simulink model "Receiver"  (R2021b)
settings: Solver=FixedStepDiscrete  StartTime=0.0  StopTime=inf  RelTol=1e-3
undefined symbols (not defined in the file): D4
libraries: androiduilib x4, androidcommunicationlib x1
settings Model: Creator=Nishikant Parmar  LastModifiedBy=Nishikant Parmar
settings OptimizationCC: EnhancedBackFolding=on  PassReuseOutputArgsAs=Individual arguments  ZeroExternalMemoryAtStartup=off  ZeroInternalMemoryAtStartup=off  MaxStackSize=64  OptimizeBlockOrder=speed  DifferentSizesBufferReuse=on  OptimizationCustomize=off  EfficientTunableParamExpr=on
settings DebuggingCC: ParameterTunabilityLossMsg=error
settings HardwareCC: ProdBitPerPointer=32  ProdBitPerSizeT=32  ProdBitPerPtrDiffT=32  ProdLargestAtomicInteger=Long  ProdLargestAtomicFloat=Double  ProdWordSize=32  ProdHWDeviceType=ARM Compatible->ARM Cortex  UseEmbeddedCoderFeatures=off  UseSimulinkCoderFeatures=off
settings SFSimCC: MATLABDynamicMemAlloc=off
settings RTWCC: Description=Embedded Coder  SystemTargetFile=ert.tlc  HardwareBoard=Android Device  TLCOptions="-aInlineSetEventsForThisBaseRateFcn=TLC_FALSE -aSuppressMultiTaskScheduler=TLC_FALSE  -aRateBasedStepFcn=0"  TemplateMakefile=ert_default_tmf  RTWVerbose=off  Toolchain=Android SDK/NDK Tools
settings CodeAppCC: ForceParamTrailComments=on  IgnoreCustomStorageClasses=off  OperatorAnnotations=on  SimulinkDataObjDesc=on  SFDataObjDesc=on  InsertBlockDesc=on
settings ERTTargetCC: SupportNonInlinedSFcns=on

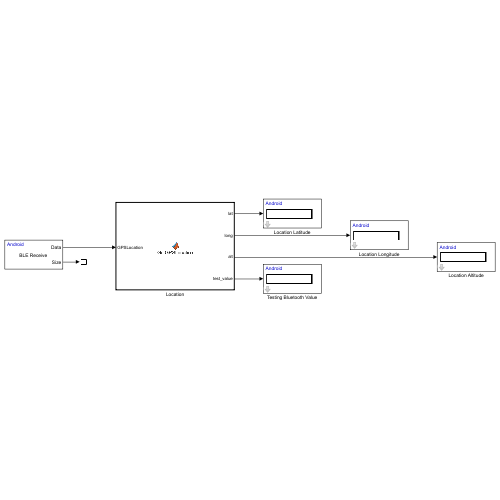
[thumbnail: Simulink's stored preview of the top-level diagram]
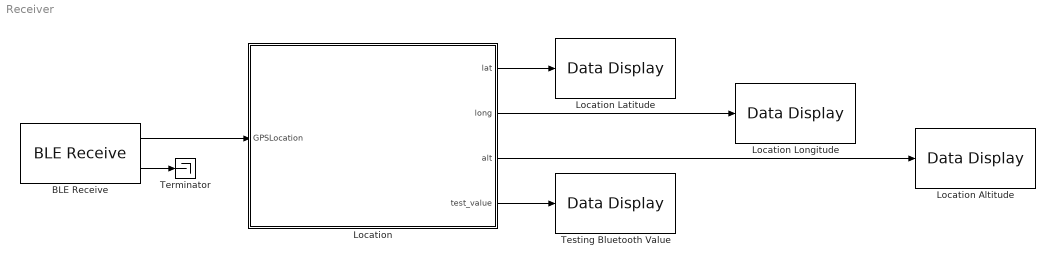
== system Receiver ==
  BLE Receive : androidcommunicationlib/BLE Receive  DeviceMode=Central (Client)  BluetoothAddress=D4:8A:39:6B:66:89  CharUUID=00002a37-0000-1000-8000-00805f9b34fb  ServiceUUID=0000180d-0000-1000-8000-00805f9b34fb  device=Nishikant's Galaxy M31s  character="Heart Rate\\Heart Rate  Measurement"  CustomService=off  ServiceName=Heart Rate  CharacteristicName="Heart Rate  Measurement"  CustomServiceUUID=<Enter Service UUID>  CustomCharUUID=<Enter Characteristic UUID>  DataSize=7  SampleTime=0.1  charseruuid=00001801-0000-1000-8000-00805f9b34fb\00002a05-0000-1000-8000-00805f9b34fb  seruuid=00001810-0000-1000-8000-00805f9b34fb  PeripheralService=0000180d-0000-1000-8000-00805f9b34fb  PeripheralCharacteristic=00002a37-0000-1000-8000-00805f9b34fb  chruuid=00002a37-0000-1000-8000-00805f9b34fb  BLEId=Receiver/BLE_Receive  Devicename=Nishikant's Galaxy M31s  IsCustomService=0
      settings: SourceProductBaseCode=ANDROID
  Location : MATLAB Function  TreatAsAtomicUnit=on
  Location Altitude : androiduilib/Data Display  DataDisplayId=Receiver/Location_Altitude  Format=Float  Precision=6  SimulateUsing=Code generation  blockPlatform=Android
      settings: SourceProductBaseCode=ANDROID
  Location Latitude : androiduilib/Data Display  DataDisplayId=Receiver/Location_Latitude  Format=Float  Precision=6  SimulateUsing=Code generation  blockPlatform=Android
      settings: SourceProductBaseCode=ANDROID
  Location Longitude : androiduilib/Data Display  DataDisplayId=Receiver/Location_Longitude  Format=Float  Precision=6  SimulateUsing=Code generation  blockPlatform=Android
      settings: SourceProductBaseCode=ANDROID
  Terminator : Terminator
  Testing Bluetooth Value : androiduilib/Data Display  DataDisplayId=Receiver/Testing_Bluetooth_Value  Format=Float  Precision=6  SimulateUsing=Code generation  blockPlatform=Android
      settings: SourceProductBaseCode=ANDROID
  wires:
  BLE Receive/2 -> Terminator/1
  BLE Receive/1 -> Location/1(GPSLocation)
  Location/1(lat) -> Location Latitude/1
  Location/2(long) -> Location Longitude/1
  Location/3(alt) -> Location Altitude/1
  Location/4(test_value) -> Testing Bluetooth Value/1

== matlab function Receiver/Location ==
  data: GPSLocation input; lat output; long output; alt output; test_value output
function [lat, long, alt, test_value] = GetGPSLocation(GPSLocation)
    

    % Convert uint8 to int8 (test_value)
    test_value_uint8 = GPSLocation(1);   
    isNegative = int8(bitget(test_value_uint8,8));
    test_value = int8(bitset(test_value_uint8,8,0)) +  (-2^7)*isNegative;    

    % Get upper and lower bits of lat, long and alt
    lower_lat=GPSLocation(2);
    upper_lat=GPSLocation(3);
    lower_long=GPSLocation(4);
    upper_long=GPSLocation(5);
    lower_alt=GPSLocation(6);
    upper_alt=GPSLocation(7); 
    

    % Combine the two halves
    lat = CombineBytes(upper_lat, lower_lat);
    long = CombineBytes(upper_long, lower_long);
    alt = CombineBytes(upper_alt, lower_alt);
end



function value = CombineBytes(upper, lower)

    % Reference - MATLAB documentation

    lower_shifted = bitshift(uint16(lower), 0);
    upper_shifted = bitshift(uint16(upper), 8);
    isNegative = int16(bitget(upper_shifted,16));
    value = int16(bitset(bitor(upper_shifted,lower_shifted),16,0)) + (-2^15)*isNegative;
end
